simulink subsystem "AUVPlant"  (R2021a)
settings: Solver=VariableStepAuto  StartTime=0.0  StopTime=10.0  RelTol=1e-3
undefined symbols (not defined in the file): dMaxX, dMaxY, dMinX, dMinY, dSeedX, dSeedY, dts, N, PWM, RPM, T200, tmax, tmin, waPhi, waPsi, waTheta, waX, waY, waZ, wfPhi, wfPsi, wfTheta, wfX, wfY, wfZ, wpPhi, wpPsi, wpTheta, wpX, wpY, wpZ
libraries: simulink x2, aerolibutil x2, dspsnks4 x1, dspvision x1, sharedtransform x1
settings Model: Creator=lamarre  LastModifiedBy=lamarre
settings SolverCC: AlgebraicLoopSolver=TrustRegion
settings DebuggingCC: SFMachineParentedDataDiag=warning

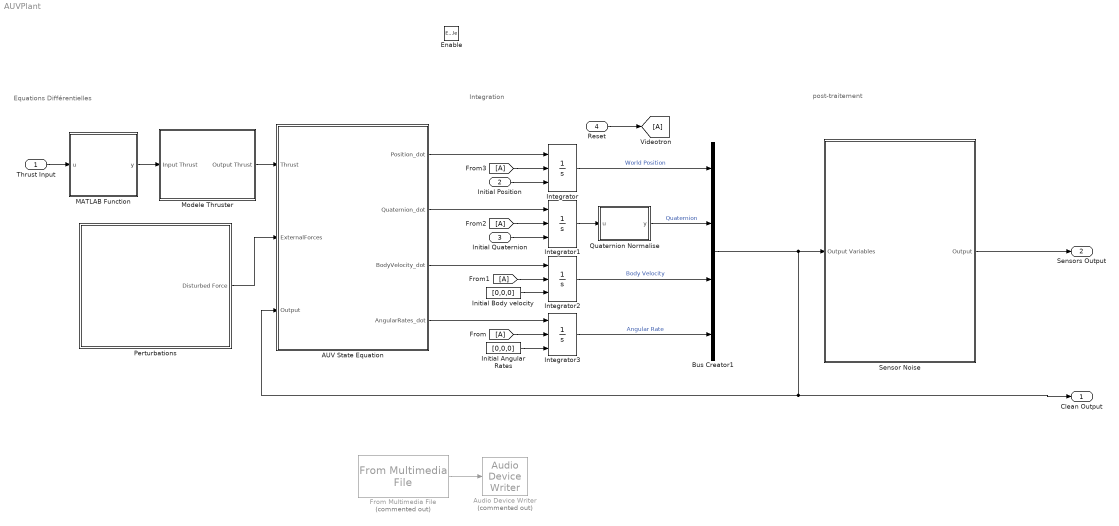
== system AUVPlant ==
  note: post-traitement
  note: Equations Différentielles
  note: Integration
  Thrust Input : Inport
  Initial Position : Inport  Port=2
  Initial Quaternion : Inport  Port=3
  Reset : Inport  Port=4
  Enable : EnablePort
  AUV State Equation : MATLAB Function  TreatAsAtomicUnit=on  SystemSampleTime=1/50
  Audio Device Writer : dspsnks4/Audio Device Writer  Commented=on  Driver=ALSA  Device=Default  InheritSampleRate=off  SampleRate=44100  BitDepth=16-bit integer  BufferSize=4096  NumBuffers=10  DefaultOutputChannelMapping=on  OutputChannelMapping=1:2  OutputNumUnderrunSamples=off  DriverIdx=8  DeviceWarnFlag=''
  Bus Creator1 : BusCreator  Inputs=4
  From Multimedia File : dspvision/From Multimedia File  Commented=on  inputFilename=warning.mp3  readRange=[1 Inf]  loop=on  numPlays=inf  outputStreams=Audio only  videoDataType=single  audioDataType=double  inheritSampleTime=off  userDefinedSampleTime=1/60  noAudioOutput=off  isIntensityVideo=off  fourcc=RGB  colorVideoFormat=Separate color signals  outputEOF=off  dataOrg=Column-major  audioFrameSize=1024  computeAudioFrameSize=off  outSamplingMode=Sample based
  Initial Angular Rates : Constant  Value=[0,0,0]
  "Initial Body velocity " : Constant  Value=[0,0,0]
  Integrator : Integrator  ExternalReset=rising  InitialConditionSource=external  InitialCondition=[0,0,1]
  Integrator1 : Integrator  ExternalReset=rising  InitialConditionSource=external  InitialCondition=[1,0,0,0]
  Integrator2 : Integrator  ExternalReset=rising  InitialConditionSource=external  InitialCondition=[0,0,0]
  Integrator3 : Integrator  ExternalReset=rising  InitialConditionSource=external  InitialCondition=[0,0,0]
  MATLAB Function : MATLAB Function  TreatAsAtomicUnit=on
  Modele Thruster : Subsystem
  Perturbations : Subsystem
  Quaternion Normalise : MATLAB Function  TreatAsAtomicUnit=on
  Sensor Noise : Subsystem
  Clean Output : Outport
  Sensors Output : Outport  Port=2
  wires:
  "Initial Body velocity "/1 -> Integrator2/3
  AUV State Equation/2(Quaternion_dot) -> Integrator1/1
  Integrator/1 -> Bus Creator1/1  "World Position"
  Integrator2/1 -> Bus Creator1/3  "Body Velocity"
  AUV State Equation/1(Position_dot) -> Integrator/1
  Initial Angular Rates/1 -> Integrator3/3
  AUV State Equation/4(AngularRates_dot) -> Integrator3/1
  Integrator3/1 -> Bus Creator1/4  "Angular Rate"
  Initial Quaternion/1 -> Integrator1/3
  AUV State Equation/3(BodyVelocity_dot) -> Integrator2/1
  [A] -> Integrator3/2
  [A] -> Integrator2/2
  [A] -> Integrator1/2
  [A] -> Integrator/2
  Initial Position/1 -> Integrator/3
  Reset/1 -> [A]
  Sensor Noise/1(Output) -> Sensors Output/1
  Modele Thruster/1(Output Thrust) -> AUV State Equation/1(Thrust)
  Bus Creator1/1 -> Sensor Noise/1(Output Variables), Clean Output/1, AUV State Equation/3(Output)
  Integrator1/1 -> Quaternion Normalise/1(u)
  Quaternion Normalise/1(y) -> Bus Creator1/2  "Quaternion"
  From Multimedia File/1 -> Audio Device Writer/1
  Thrust Input/1 -> MATLAB Function/1(u)
  MATLAB Function/1(y) -> Modele Thruster/1(Input Thrust)
  Perturbations/1(Disturbed Force) -> AUV State Equation/2(ExternalForces)

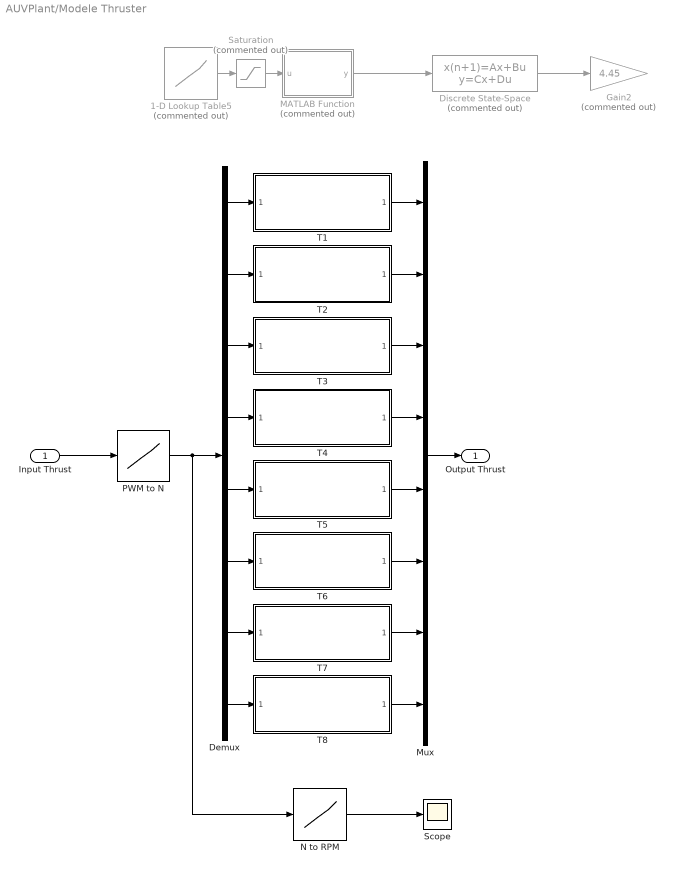
== system AUVPlant/Modele Thruster ==
  Input Thrust : Inport
  " PWM to N" : Lookup_n-D  NumberOfTableDimensions=1  BreakpointsForDimension1=PWM  BreakpointsForDimension1DataTypeStr=uint16  BeginIndexSearchUsingPreviousIndexResult=on  Table=N  TableDataTypeStr=double  InterpMethod=Nearest  ExtrapMethod=Clip  InternalRulePriority=Speed  OutDataTypeStr=double  RndMeth=Simplest  InputSameDT=on
  1-D Lookup Table5 : Lookup_n-D  Commented=on  NumberOfTableDimensions=1  BreakpointsForDimension1=N  Table=PWM  InterpMethod=Nearest  InternalRulePriority=Speed  RndMeth=Simplest  InputSameDT=on
  Demux : Demux  Outputs=8
  Discrete State-Space : DiscreteStateSpace  Commented=on  A=T200.A  B=T200.B  C=T200.C  D=T200.D  SampleTime=T200.Ts
  Gain2 : Gain  Commented=on  Gain=4.45
  MATLAB Function : MATLAB Function  Commented=on  TreatAsAtomicUnit=on
  Mux : Mux  Inputs=8
  N to RPM : Lookup_n-D  NumberOfTableDimensions=1  BreakpointsForDimension1=N  BreakpointsForDimension1DataTypeStr=double  BeginIndexSearchUsingPreviousIndexResult=on  Table=RPM  TableDataTypeStr=double  InterpMethod=Nearest  ExtrapMethod=Clip  InternalRulePriority=Speed  OutDataTypeStr=uint16  RndMeth=Simplest  InputSameDT=on
  Saturation : Saturate  Commented=on  UpperLimit=tmax  LowerLimit=tmin  LinearizeAsGain=off  ZeroCross=off
  Scope : Scope
  T{1..8} (8 alike) : Subsystem  ReferencedSubsystem=ThrusterModel
  Output Thrust : Outport
  wires:
  N to RPM/1 -> Scope/1
  Input Thrust/1 -> " PWM to N"/1
  " PWM to N"/1 -> Demux/1, N to RPM/1
  Saturation/1 -> MATLAB Function/1(u)
  1-D Lookup Table5/1 -> Saturation/1
  Discrete State-Space/1 -> Gain2/1
  MATLAB Function/1(y) -> Discrete State-Space/1
  Demux/1 -> T1/1
  Demux/2 -> T2/1
  Demux/3 -> T3/1
  Demux/4 -> T4/1
  Demux/5 -> T5/1
  Demux/6 -> T6/1
  Demux/8 -> T8/1
  Demux/7 -> T7/1
  T1/1 -> Mux/1
  T2/1 -> Mux/2
  T3/1 -> Mux/3
  T4/1 -> Mux/4
  T5/1 -> Mux/5
  T6/1 -> Mux/6
  T7/1 -> Mux/7
  T8/1 -> Mux/8
  Mux/1 -> Output Thrust/1

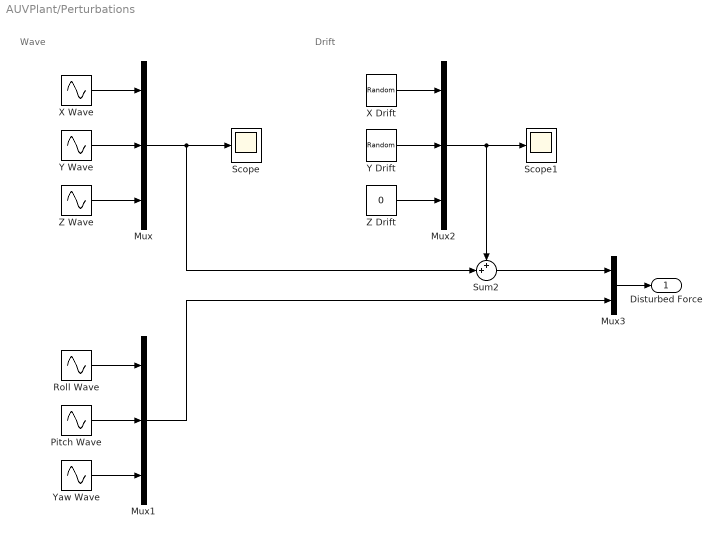
== system AUVPlant/Perturbations ==
  note: Drift
  note: Wave
  Mux : Mux  Inputs=3
  Mux1 : Mux  Inputs=3
  Mux2 : Mux  Inputs=3
  Mux3 : Mux  Inputs=2
  Pitch Wave : Sin  Amplitude=waTheta  Frequency=wfTheta  Phase=wpTheta  SampleTime=0
  Roll Wave : Sin  Amplitude=waPhi  Frequency=wfPhi  Phase=wpPhi  SampleTime=0
  Scope : Scope
  Scope1 : Scope
  Sum2 : Sum  Inputs=++|
  X Drift : UniformRandomNumber  Minimum=dMinX  Maximum=dMaxX  Seed=dSeedX  SampleTime=dts
  X Wave : Sin  Amplitude=waX  Frequency=wfX  Phase=wpX  SampleTime=0
  Y Drift : UniformRandomNumber  Minimum=dMinY  Maximum=dMaxY  Seed=dSeedY  SampleTime=dts
  Y Wave : Sin  Amplitude=waY  Frequency=wfY  Phase=wpY  SampleTime=0
  Yaw Wave : Sin  Amplitude=waPsi  Frequency=wfPsi  Phase=wpPsi  SampleTime=0
  Z Drift : Constant  Value=0
  Z Wave : Sin  Amplitude=waZ  Frequency=wfZ  Phase=wpZ  SampleTime=0
  Disturbed Force : Outport
  wires:
  Roll Wave/1 -> Mux1/1
  Pitch Wave/1 -> Mux1/2
  Mux3/1 -> Disturbed Force/1
  Sum2/1 -> Mux3/1
  X Wave/1 -> Mux/1
  Y Wave/1 -> Mux/2
  Z Wave/1 -> Mux/3
  Yaw Wave/1 -> Mux1/3
  Mux1/1 -> Mux3/2
  Mux2/1 -> Scope1/1, Sum2/1
  X Drift/1 -> Mux2/1
  Y Drift/1 -> Mux2/2
  Mux/1 -> Sum2/2, Scope/1
  Z Drift/1 -> Mux2/3

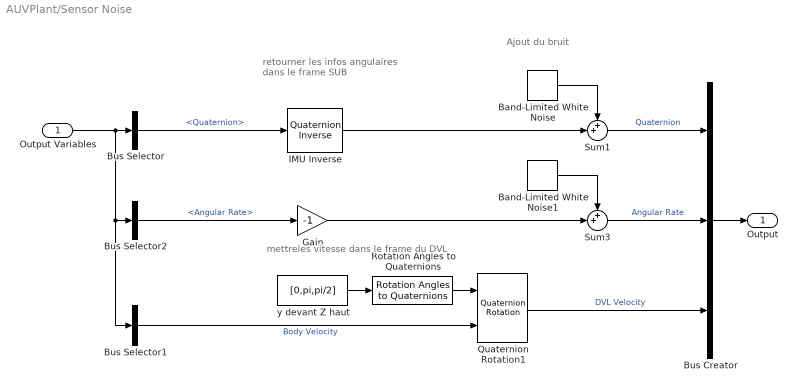
== system AUVPlant/Sensor Noise ==
  note: retourner les infos
      | angulaires dans
      | le frame SUB
  note: mettreles vitesse dans le frame du DVL
  note: Ajout du bruit
  Output Variables : Inport
  " y devant Z haut" : Constant  Value=[0,pi,pi/2]
  Band-Limited White Noise : simulink/Sources/Band-Limited White Noise  Cov=[0.00000000025]  Ts=1/100  seed=[23341]
  Band-Limited White Noise1 : simulink/Sources/Band-Limited White Noise  Cov=[0.0000000004]  Ts=1/100  seed=[23341]
  Bus Creator : BusCreator  Inputs=3
  Bus Selector : BusSelector  OutputSignals=Quaternion
  Bus Selector1 : BusSelector  OutputSignals=Body Velocity  OutputAsBus=on
  Bus Selector2 : BusSelector  OutputSignals=Angular Rate
  Gain : Gain  Gain=-1
  IMU Inverse : aerolibutil/Quaternion Inverse
  Quaternion Rotation1 : aerolibutil/Quaternion Rotation
  Rotation Angles to Quaternions : sharedtransform/Rotation Angles to Quaternions  rotationOrder=XYZ  aMode=aMode
      settings: SourceProductBaseCode=AE,PW,MT,VE,VP
  Sum1 : Sum  Inputs=++|
  Sum3 : Sum  Inputs=++|
  Output : Outport
  wires:
  Band-Limited White Noise/1 -> Sum1/1
  IMU Inverse/1 -> Sum1/2
  Gain/1 -> Sum3/2
  Rotation Angles to Quaternions/1 -> Quaternion Rotation1/1
  Bus Selector1/1 -> Quaternion Rotation1/2  "Body Velocity"
  Quaternion Rotation1/1 -> Bus Creator/3  "DVL Velocity"
  " y devant Z haut"/1 -> Rotation Angles to Quaternions/1
  Sum3/1 -> Bus Creator/2  "Angular Rate"
  Sum1/1 -> Bus Creator/1  "Quaternion"
  Band-Limited White Noise1/1 -> Sum3/1
  Bus Selector2/1 -> Gain/1  "<Angular Rate>"
  Bus Creator/1 -> Output/1
  Bus Selector/1 -> IMU Inverse/1  "<Quaternion>"
  Output Variables/1 -> Bus Selector/1, Bus Selector1/1, Bus Selector2/1

== matlab function AUVPlant/AUV State Equation ==
  data: Thrust input; ExternalForces input; Output input; Position_dot output size=3; Quaternion_dot output size=4; BodyVelocity_dot output size=3; AngularRates_dot output size=3
function [Position_dot,Quaternion_dot,BodyVelocity_dot, AngularRates_dot] = AUVStateEquation(Thrust,ExternalForces,Output)

Dynamics=AUVQuatPerturbedSimFcn(Output,ExternalForces,Thrust);

Position_dot=Dynamics(1:3);
Quaternion_dot = Dynamics(4:7);
BodyVelocity_dot= Dynamics(8:10);
AngularRates_dot = Dynamics(11:13);

== matlab function AUVPlant/MATLAB Function ==
  data: u input; y output
function y = wrapPWM(u)
 for i=1: size(u,1)
     if u(i)<1100 || u(i)>1900
         u(i)=1500;
     end
 end
y = u;

== matlab function AUVPlant/Modele Thruster/MATLAB Function ==
  data: u input; y output
function y = fcn(u)
pwm=u-1500;
if pwm>=0 
    y=pwm;
else
   y=pwm*0.77969348659;
end

== matlab function AUVPlant/Quaternion Normalise ==
  data: u input size=4; y output size=4
function y = Normalize(u)
%Normailse le quaternions pour éviter la distortions crée par l'erreur de
% de l'intégration.
d=norm(u);
y = u/d;
